simulink model "MEDOUP"  (R2022b)
settings: configuration reference "SharedConfig" (kept outside this file)
values from neighbouring files (symbols this model uses):
  McuData1DaDialEna_C = 0.0    [MEDOUP.sldd]
  McuData1DaDialVal_CA : value not decoded    [MEDOUP.sldd]
undefined symbols (not defined in the file or in its folder): slcm
libraries: canmsglib x1
Description:
  | Converts engineering unit signals into raw outputs for the medium rate task.
settings Model: DataDictionary=MEDOUP.sldd  Creator=Kevin  LastModifiedBy=Max Kolesnikov
settings ConfigSetRef: SourceName=SharedConfig

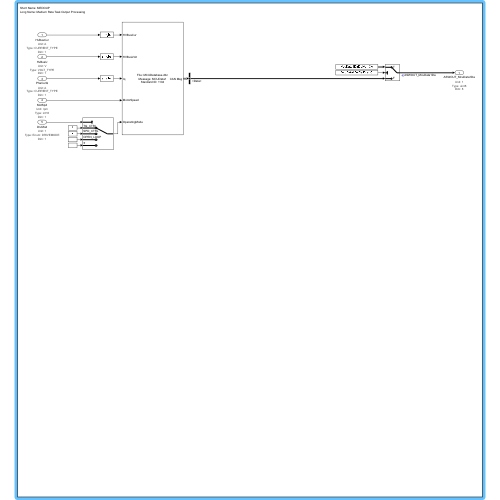
[thumbnail: Simulink's stored preview of the top-level diagram]
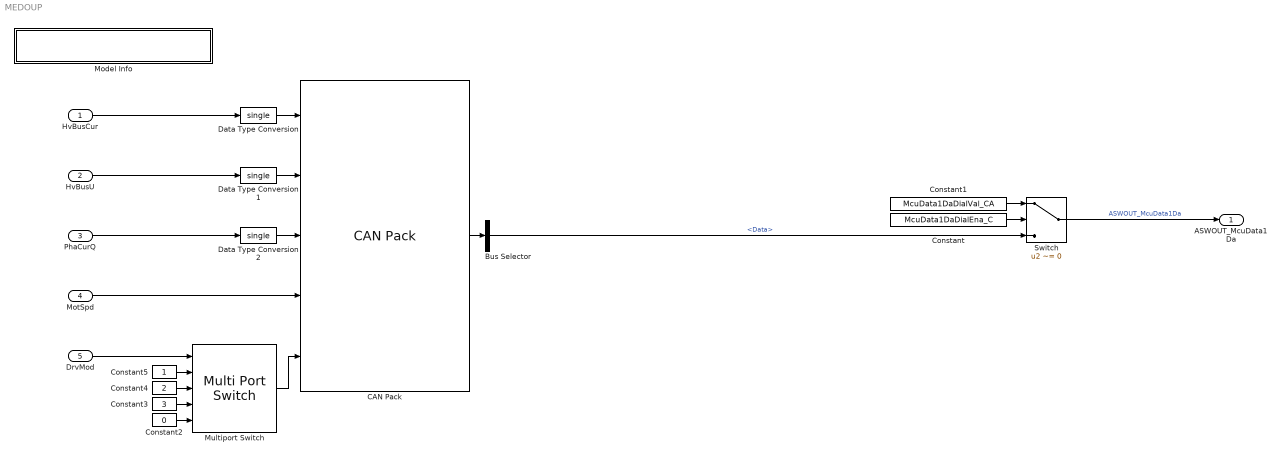
== system MEDOUP ==
  HvBusCur : Inport  OutDataTypeStr=CURRENT_TYPE  Unit=A  PortDimensions=1
      settings: AttributesFormatString=|
      | Unit: %<Unit>
      | Type: %<OutDataTypeStr>
      | Dim: %<PortDimensions>
  HvBusU : Inport  Port=2  OutDataTypeStr=VOLT_TYPE  Unit=V  PortDimensions=1
      settings: AttributesFormatString=|
      | Unit: %<Unit>
      | Type: %<OutDataTypeStr>
      | Dim: %<PortDimensions>
  PhaCurQ : Inport  Port=3  OutDataTypeStr=CURRENT_TYPE  Unit=A  PortDimensions=1
      settings: AttributesFormatString=|
      | Unit: %<Unit>
      | Type: %<OutDataTypeStr>
      | Dim: %<PortDimensions>
  MotSpd : Inport  Port=4  OutDataTypeStr=int16  Unit=rpm  PortDimensions=1
      settings: AttributesFormatString=|
      | Unit: %<Unit>
      | Type: %<OutDataTypeStr>
      | Dim: %<PortDimensions>
  DrvMod : Inport  Port=5  OutDataTypeStr=Enum: DRIVEMODE  Unit=1  PortDimensions=1
      settings: AttributesFormatString=|
      | Unit: %<Unit>
      | Type: %<OutDataTypeStr>
      | Dim: %<PortDimensions>
  Bus Selector : BusSelector  OutputSignals=Data
  CAN Pack : canmsglib/CAN Pack  CANdbFile=C:\MKSTechRepos\P2319\p2319asw01\asw\lib\MCUDatabase.dbc  MsgList=MCUData1  MsgName=MCUData1  MsgIDType=Standard (11-bit identifier)  MsgIdentifier=1104  MsgLength=8  Remote=off  ApplyMinMax=off  BusOutput=on  SignalInfo={'HVBusCur','16','16','LE','unsigned','Standard','0','0.02','-650','-650','660.7';'HVBusVolt','0','12','LE','unsigned','Standard','0','0.1','0','0','409.5';'Iq','32','16','LE','unsigned','Standard','0','0.02','-650','-650','660.7';'MotorSpeed','48','16','LE','unsigned','Standard','0','1','-32500','-32500','33035';'OperatingMode','12','2','LE','unsigned','Standard','0','1','0','-Inf','Inf'}
      settings: LibrarySourceBlock=embeddedtargetslib/Host Communication/CAN Pack  DataFormat=CANdb specified signals
  Constant : Constant  Value=McuData1DaDialEna_C
  Constant1 : Constant  Value=McuData1DaDialVal_CA
  Constant2 : Constant  Value=0  OutDataTypeStr=uint8
  Constant3 : Constant  Value=3  OutDataTypeStr=uint8
  Constant4 : Constant  Value=2  OutDataTypeStr=uint8
  Constant5 : Constant  OutDataTypeStr=uint8
  Data Type Conversion : DataTypeConversion  OutDataTypeStr=single  SaturateOnIntegerOverflow=off  RndMeth=Floor
  Data Type Conversion1 : DataTypeConversion  OutDataTypeStr=single  SaturateOnIntegerOverflow=off  RndMeth=Floor
  Data Type Conversion2 : DataTypeConversion  OutDataTypeStr=single  SaturateOnIntegerOverflow=off  RndMeth=Floor
  Model Info : Subsystem  LoadFcn=slcm LoadBlock;  InitFcn=slcm('UpdateAllCMBlocksInThisModelInit')  mask(CMBlock){Frame=off, DisplayStringWithTags=|, MaskDisplayString=Short Name: MEDOUP\nLong Name: Medium Rate Task Output Processing, HorizontalTextAlignment=Left, LeftAlignmentValue=0.02}
      mask DisplayStringWithTags=|
      | Short Name: %<ModelName>
      | Long Name: Medium Rate Task Output Processing
      mask prompts: Frame "Simulink:masks:Frame_MP"; DisplayStringWithTags "Simulink:masks:DisplayStringWithTags_MP"; MaskDisplayString "Simulink:masks:MaskDisplayString_MP"; HorizontalTextAlignment "Simulink:masks:HorizontalTextAlignment_MP"; LeftAlignmentValue "Simulink:masks:LeftAlignmentValue_MP"
      mask help: Simulink:masks:CMBlock_MD
      settings: CopyFcn=slcm CopyBlock;  DeleteFcn=slcm Cancel;  PostSaveFcn=slcm('UpdateAllCMBlocksInThisModel')  NameChangeFcn=slcm Rename;  OpenFcn=slcm
      mask Display: text(slResolve(LeftAlignmentValue, gcbh), 0.5, MaskDisplayString, 'HorizontalAlignment', HorizontalTextAlignment)
  Multiport Switch : MultiPortSwitch  DataPortOrder=Specify indices  DataPortIndices={DRIVEMODE.TQ_CTRL,DRIVEMODE.SPD_CTRL,DRIVEMODE.OPEN_LOOP}  DataPortForDefault=Additional data port  DiagnosticForDefault=None  SaturateOnIntegerOverflow=off  InputSameDT=off
  Switch : Switch  Criteria=u2 ~= 0  SaturateOnIntegerOverflow=off  InputSameDT=off
  ASWOUT_McuData1Da : Outport  OutDataTypeStr=uint8  Unit=1  PortDimensions=8
      settings: AttributesFormatString=|
      | Unit: %<Unit>
      | Type: %<OutDataTypeStr>
      | Dim: %<PortDimensions>
  wires:
  Switch/1 -> ASWOUT_McuData1Da/1  "ASWOUT_McuData1Da"
  CAN Pack/1 -> Bus Selector/1
  Constant1/1 -> Switch/1
  Constant/1 -> Switch/2
  Bus Selector/1 -> Switch/3  "<Data>"
  HvBusCur/1 -> Data Type Conversion/1
  HvBusU/1 -> Data Type Conversion1/1
  PhaCurQ/1 -> Data Type Conversion2/1
  MotSpd/1 -> CAN Pack/4
  DrvMod/1 -> Multiport Switch/1
  Multiport Switch/1 -> CAN Pack/5
  Constant2/1 -> Multiport Switch/5
  Constant5/1 -> Multiport Switch/2
  Constant4/1 -> Multiport Switch/3
  Constant3/1 -> Multiport Switch/4
  Data Type Conversion/1 -> CAN Pack/1
  Data Type Conversion1/1 -> CAN Pack/2
  Data Type Conversion2/1 -> CAN Pack/3

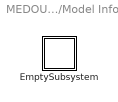
== system MEDOUP/Model Info ==
  EmptySubsystem : Subsystem

== system MEDOUP/Model Info/EmptySubsystem ==
